simulink model "calculate_collision_effects"  (R2018a)
settings: Solver=VariableStepAuto  StartTime=0.0  StopTime=120  FixedStep=0.01  MaxStep=.01  RelTol=1e-3
values from neighbouring files (symbols this model uses):
  collision_detection_distance = 2    [params.mat]
  push_force = 5    [params.mat]
settings Model: Creator=U500304  LastModifiedBy=U500304
settings SolverCC: ZeroCrossAlgorithm=Adaptive
settings DataIOCC: SaveOutput=off  SaveTime=off
settings DebuggingCC: MaxConsecutiveZCsMsg=warning

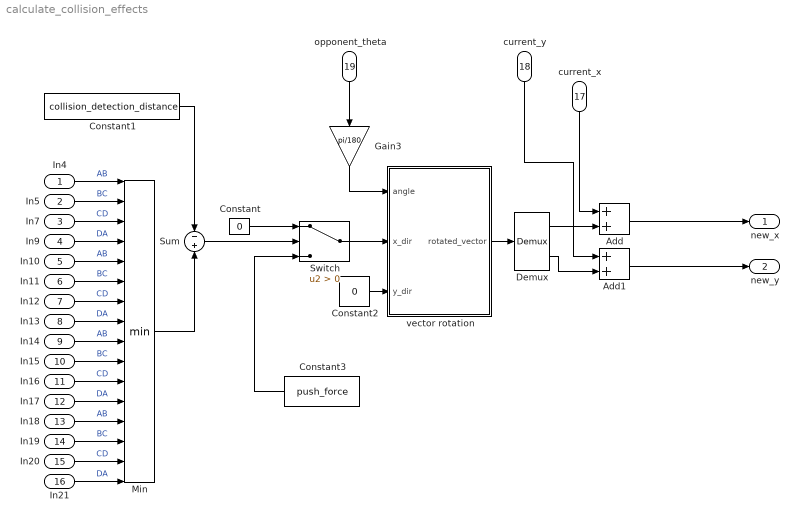
== system calculate_collision_effects ==
  In4 : Inport  OutDataTypeStr=double  PortDimensions=1  SampleTime=0
  In5 : Inport  Port=2  OutDataTypeStr=double  PortDimensions=1  SampleTime=0
  In7 : Inport  Port=3  OutDataTypeStr=double  PortDimensions=1  SampleTime=0
  In9 : Inport  Port=4  OutDataTypeStr=double  PortDimensions=1  SampleTime=0
  In10 : Inport  Port=5  OutDataTypeStr=double  PortDimensions=1  SampleTime=0
  In11 : Inport  Port=6  OutDataTypeStr=double  PortDimensions=1  SampleTime=0
  In12 : Inport  Port=7  OutDataTypeStr=double  PortDimensions=1  SampleTime=0
  In13 : Inport  Port=8  OutDataTypeStr=double  PortDimensions=1  SampleTime=0
  In14 : Inport  Port=9  OutDataTypeStr=double  PortDimensions=1  SampleTime=0
  In15 : Inport  Port=10  OutDataTypeStr=double  PortDimensions=1  SampleTime=0
  In16 : Inport  Port=11  OutDataTypeStr=double  PortDimensions=1  SampleTime=0
  In17 : Inport  Port=12  OutDataTypeStr=double  PortDimensions=1  SampleTime=0
  In18 : Inport  Port=13  OutDataTypeStr=double  PortDimensions=1  SampleTime=0
  In19 : Inport  Port=14  OutDataTypeStr=double  PortDimensions=1  SampleTime=0
  In20 : Inport  Port=15  OutDataTypeStr=double  PortDimensions=1  SampleTime=0
  In21 : Inport  Port=16  OutDataTypeStr=double  PortDimensions=1  SampleTime=0
  current_x : Inport  Port=17  OutDataTypeStr=double  PortDimensions=1  SampleTime=0
  current_y : Inport  Port=18  OutDataTypeStr=double  PortDimensions=1  SampleTime=0
  opponent_theta : Inport  Port=19  OutDataTypeStr=double  PortDimensions=1  SampleTime=0
  Add : Sum
  Add1 : Sum
  Constant : Constant  Value=0
  Constant1 : Constant  Value=collision_detection_distance
  Constant2 : Constant  Value=0
  Constant3 : Constant  Value=push_force
  Demux : Demux  Outputs=2
  Gain3 : Gain  Gain=pi/180
  Min : MinMax  Inputs=16
  Sum : Sum  Inputs=-+
  Switch : Switch  Criteria=u2 > Threshold
  "vector rotation " : Subsystem
  new_x : Outport  OutDataTypeStr=double  PortDimensions=1  SampleTime=0
  new_y : Outport  Port=2  OutDataTypeStr=double  PortDimensions=1  SampleTime=0
  wires:
  "vector rotation "/1("rotated_vector ") -> Demux/1
  Min/1 -> Sum/2
  In17/1 -> Min/12  "DA"
  Constant2/1 -> "vector rotation "/3(y_dir)
  Demux/1 -> Add/2
  Gain3/1 -> "vector rotation "/1(angle)
  current_y/1 -> Add1/1
  In4/1 -> Min/1  "AB"
  Constant3/1 -> Switch/3
  current_x/1 -> Add/1
  In19/1 -> Min/14  "BC"
  Switch/1 -> "vector rotation "/2(x_dir)
  Demux/2 -> Add1/2
  In10/1 -> Min/5  "AB"
  In11/1 -> Min/6  "BC"
  In16/1 -> Min/11  "CD"
  In12/1 -> Min/7  "CD"
  In9/1 -> Min/4  "DA"
  In15/1 -> Min/10  "BC"
  Add/1 -> new_x/1
  In13/1 -> Min/8  "DA"
  In18/1 -> Min/13  "AB"
  In7/1 -> Min/3  "CD"
  Add1/1 -> new_y/1
  In14/1 -> Min/9  "AB"
  opponent_theta/1 -> Gain3/1
  In5/1 -> Min/2  "BC"
  In20/1 -> Min/15  "CD"
  In21/1 -> Min/16  "DA"
  Constant/1 -> Switch/1
  Constant1/1 -> Sum/1
  Sum/1 -> Switch/2

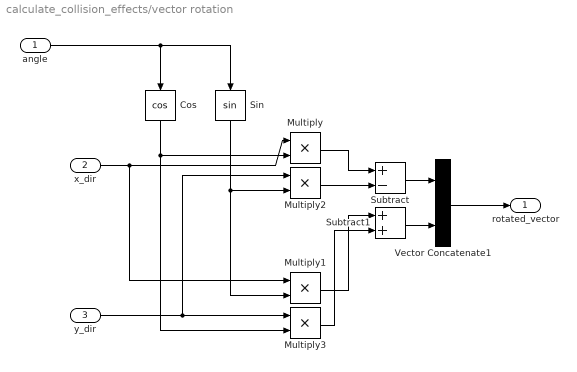
== system calculate_collision_effects/vector rotation  ==
  angle : Inport
  x_dir : Inport  Port=2
  y_dir : Inport  Port=3
  Cos : Trigonometry  Operator=cos
  Multiply{,1..3} (4 alike) : Product
  Sin : Trigonometry
  Subtract : Sum  Inputs=+-
  Subtract1 : Sum
  Vector Concatenate1 : Concatenate
  "rotated_vector " : Outport
  wires:
  Multiply3/1 -> Subtract1/2
  Multiply1/1 -> Subtract1/1
  Multiply/1 -> Subtract/1
  y_dir/1 -> Multiply3/1, Multiply2/1
  Subtract1/1 -> Vector Concatenate1/2
  Cos/1 -> Multiply3/2, Multiply/2
  Sin/1 -> Multiply1/2, Multiply2/2
  angle/1 -> Cos/1, Sin/1
  x_dir/1 -> Multiply1/1, Multiply/1
  Vector Concatenate1/1 -> "rotated_vector "/1
  Subtract/1 -> Vector Concatenate1/1
  Multiply2/1 -> Subtract/2
